simulink model "boatx010"  (R2019b)
settings: Solver=ode4  StartTime=0.0  StopTime=20  FixedStep=0.01  RelTol=1e-3  EnableMultiTasking=on
values from neighbouring files (symbols this model uses):
  A = 10    [sm_boat_runx010.m]
  a1 = a1n(nx)    [sm_boat_runx010.m]
  a2 = a2n(nx)    [sm_boat_runx010.m]
  a3 = a3n(nx)    [sm_boat_runx010.m]
  aa = 50    [sm_boat_runx010.m]
  B = 10    [sm_boat_runx010.m]
  bmax = pi*(0.47)    (= 1.47654854719)    [sm_boat_runx010.m]
  d1 = d1n(nx)    [sm_boat_runx010.m]
  d2 = d2n(nx)    [sm_boat_runx010.m]
  d3 = d3n(nx)    [sm_boat_runx010.m]
  fixedstep = 0.01    [sm_boat_runx010.m]
  Fmax = 20    [sm_boat_runx010.m]
  H = 0.20    (= 0.2)    [sm_boat_runx010.m]
  Iz = m*(W^2+L^2)/12    (= 0.759791666667)    [sm_boat_runx010.m]
  Izz = (0.1*m*W^2+1000*pi*D^2*L^3)/2/12    (= 0.336072151416)    [sm_boat_runx010.m]
  kai = pi*2/8    (= 0.785398163397)    [sm_boat_runx010.m]
  L = 1    [sm_boat_runx010.m]
  Lt = 0.4    [sm_boat_runx010.m]
  m = 7    [sm_boat_runx010.m]
  mxx = 0.05*m    (= 0.35)    [sm_boat_runx010.m]
  myy = 1000*pi*D^2*L/2    (= 3.92699081699)    [sm_boat_runx010.m]
  n_o_w = length(wps)    [sm_boat_runx010.m]
  td = 0    [sm_boat_runx010.m]
  W = 0.55    [sm_boat_runx010.m]
  wd = fd*2*pi    (= 0.628318530718)    [sm_boat_runx010.m]
  wp_sh = 10    [sm_boat_runx010.m]
  wp_tol = 1    [sm_boat_runx010.m]
  wps = [0 0; -aa -aa; aa -aa; aa/2 -aa/2; aa/2 aa/2; aa aa; -aa aa; -aa/2 aa/2; -aa/2 0; -aa/5 0]    [sm_boat_runx010.m]
undefined symbols (not defined in the file or in its folder): X, Y, Z
libraries: sm_lib x36, nesl_utility x11
(part 1 of 2)
settings Model: Creator=huangy  LastModifiedBy=ya
settings DataIOCC: LimitDataPoints=on  SaveFormat=Array  ReturnWorkspaceOutputs=off
settings OptimizationCC: LifeSpan=inf
settings DebuggingCC: SFUnexpectedBacktrackingDiag=warning  SFNoUnconditionalDefaultTransitionDiag=warning  ArithmeticOperatorsInVariantConditions=warning
settings HardwareCC: ProdBitPerPointer=32  ProdBitPerSizeT=32  ProdBitPerPtrDiffT=32  ProdLargestAtomicFloat=None  ProdIntDivRoundTo=Undefined  ProdEndianess=Unspecified  ProdWordSize=32  ProdHWDeviceType=32-bit Generic
settings ModelReferenceCC: PropagateSignalLabelsOutOfModel=off
settings SFSimCC: SimUseLocalCustomCode=off  CustomCodeUndefinedFunction=UseInterfaceOnly
settings RTWCC: RTWUseLocalCustomCode=off
settings CodeAppCC: StateflowObjectComments=on
settings GRTTargetCC: TargetLangStandard=C89/C90 (ANSI)  GeneratePreprocessorConditionals=Disable all
settings ConfigComp: CovMetricSettings=dw  CovHtmlReporting=on  CovSaveCumulativeToWorkspaceVar=on  CovSaveSingleToWorkspaceVar=on  CovExternalEMLEnable=off
settings SimscapeCC: SimscapeNormalizeSystem=off
settings ConfigurationSet: Description=SimMechanics 2G
settings ExplorerConfigSet: InternalSimMechanicsExplorerSettings="<ExplorerConfiguration><canonicalview>default</canonicalview><AnimationSetting><BasePlaybackSpeed>1.0</BasePlaybackSpeed><PlaybackSpeedFactor>1.0</PlaybackSpeedFactor></AnimationSetting><TilePanel><TileInfo><Tiles Columns=\"1\" Count=\"1\" Rows=\"1\"><Column Weight=\"1\"/><Row Weight=\"1\"/><Tile Height=\"1\" Width=\"1\" X=\"0\" Y=\"0\"/></Tiles></TileInfo><SceneInfo><SceneViewer><BGColor><R>0.60000002384185791</R><G>0.60000002384185791</G><B>0.60000002384185791</B></BGColor><Camera><DoPerspective>off</DoPerspective><Position><X>40.4002730296998891</X><Y>-86.2507379862350376</Y><Z>44.8685618917037345</Z></Position><Center><X>-16.7562514385694357</X><Y>-29.0942135179657271</Y><Z>-12.2879625765655653</Z></Center><Up><X>-0.408248290463863073</X><Y>0.408248290463863073</Y><Z>0.816496580927726145</Z></Up><ViewLimDist>1</ViewLimDist><YLim>29.9592729600567189</YLim><XLim>38.3059771851572677</XLim></Camera></SceneViewer></SceneInfo></TilePanel><MechEditorPanel><Cameras/><GfxPanelCameraMap/><VideoCreator><PlaybackSpeedRatio>1.0</PlaybackSpeedRatio><FrameRate>30</FrameRate><VideoFormat>MPEG-4</VideoFormat><FrameSize>[800 600]</FrameSize></VideoCreator></MechEditorPanel></ExplorerConfiguration>"

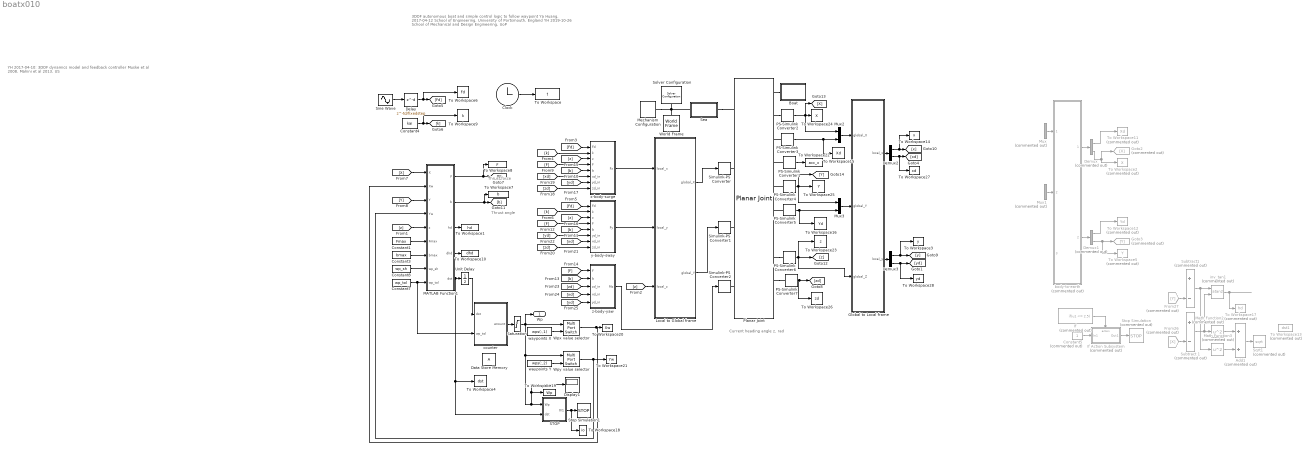
== system boatx010 ==
  note: 3DOF autonomous boat and simple control logic to follow waypoint
      | Ya Huang, 2017-04-12 School of Engineering, University of Portsmouth, England
      | YH 2019-10-26 School of Mechanical and Design Engineering, UoP
  note: Thrust force
  note: Thrust angle
  note: Current heading angle z, rad
  note: YH 2017-04-10:
      | 3DOF dynamics model and feedback controller
      | Muske et al 2008, Mahini et al 2013, US
  Add1 : Sum  Commented=on
  Boat : Subsystem  mask{d=L, w=W, h=H, m=m, Iz=Iz}
      mask prompts: d "Depth d (m)"; w "Width w (m)"; h "Height h (m)"; m "Mass m (kg)"; Iz "Mass moent of inertia"
  Clock : Clock
  Constant1 : Constant  Value=Fmax  VectorParams1D=off
  Constant3 : Constant  Value=bmax  VectorParams1D=off
  Constant4 : Constant  Value=kai
  Constant5 : Constant  Commented=on  VectorParams1D=off
  Constant7 : Constant  Value=wp_tol  VectorParams1D=off
  Constant8 : Constant  Value=wp_sh  VectorParams1D=off
  Data Store Memory : DataStoreMemory  ReadBeforeWriteMsg=warning  WriteAfterWriteMsg=warning  WriteAfterReadMsg=warning  ShowAdditionalParam=off  OutDataTypeStr=single
  Delay : Delay  DelayLength=td/fixedstep  InitialCondition=0
  Demux : Demux  Commented=on  Outputs=2
  Demux1 : Demux  Commented=on  Outputs=2
  Demux2 : Demux  Outputs=2
  Demux3 : Demux  Outputs=2
  Display1 : Display
  From26 : From  Commented=on  GotoTag=X
  From27 : From  Commented=on  GotoTag=Y
  Global to Local frame : Subsystem
  Goto2 : Goto  Commented=on  GotoTag=X
  Goto3 : Goto  Commented=on  GotoTag=Y
  If : If  Commented=on  IfExpression=u1 <= 2.5  ShowElse=off
  If Action Subsystem : Subsystem  Commented=on  TreatAsAtomicUnit=on
  Local to Global frame : Subsystem
  MATLAB Function1 : MATLAB Function  TreatAsAtomicUnit=on
  Math Function2 : Math  Commented=on  Operator=square  SaturateOnIntegerOverflow=on
  Math Function3 : Math  Commented=on  Operator=square  SaturateOnIntegerOverflow=on
  Mechanism Configuration : sm_lib/Utilities/Mechanism Configuration  UniformGravity=Constant  GravityVector=[0 0 -9.80665]  GravityUnits=m/s^2  LinearizationDelta=0.001
  Mux : Mux  Commented=on  Inputs=2
  Mux1 : Mux  Commented=on  Inputs=2
  Mux2 : Mux  Inputs=2
  Mux3 : Mux  Inputs=2
  PS-Simulink Converter1 : nesl_utility/PS-Simulink Converter  PhysicalDomain=network_engine_domain  SubClassName=ps_output  LeftPortType=input  RightPortType=output  PseudoPeriodic=off  Frequencies=[]  Unit=m/s^2  AffineConversion=off
  PS-Simulink Converter2 : nesl_utility/PS-Simulink Converter  PhysicalDomain=network_engine_domain  SubClassName=ps_output  LeftPortType=input  RightPortType=output  PseudoPeriodic=off  Frequencies=[]  Unit=m  AffineConversion=off
  PS-Simulink Converter3 : nesl_utility/PS-Simulink Converter  PhysicalDomain=network_engine_domain  SubClassName=ps_output  LeftPortType=input  RightPortType=output  PseudoPeriodic=off  Frequencies=[]  Unit=m/s  AffineConversion=off
  PS-Simulink Converter4 : nesl_utility/PS-Simulink Converter  PhysicalDomain=network_engine_domain  SubClassName=ps_output  LeftPortType=input  RightPortType=output  PseudoPeriodic=off  Frequencies=[]  Unit=m  AffineConversion=off
  PS-Simulink Converter5 : nesl_utility/PS-Simulink Converter  PhysicalDomain=network_engine_domain  SubClassName=ps_output  LeftPortType=input  RightPortType=output  PseudoPeriodic=off  Frequencies=[]  Unit=m/s  AffineConversion=off
  PS-Simulink Converter6 : nesl_utility/PS-Simulink Converter  PhysicalDomain=network_engine_domain  SubClassName=ps_output  LeftPortType=input  RightPortType=output  PseudoPeriodic=off  Frequencies=[]  Unit=rad  AffineConversion=off
  PS-Simulink Converter7 : nesl_utility/PS-Simulink Converter  PhysicalDomain=network_engine_domain  SubClassName=ps_output  LeftPortType=input  RightPortType=output  PseudoPeriodic=off  Frequencies=[]  Unit=rad/s  AffineConversion=off
  Planar Joint : sm_lib/Joints/Planar Joint  JointMode=Normal  SenseConstraintForce=off  SenseConstraintForceX=off  SenseConstraintForceY=off  SenseConstraintForceZ=off  SenseConstraintTorque=off  SenseConstraintTorqueX=off  SenseConstraintTorqueY=off  SenseConstraintTorqueZ=off  SenseTotalForce=off  SenseTotalForceX=off  SenseTotalForceY=off  SenseTotalForceZ=off  SenseTotalTorque=off  SenseTotalTorqueX=off  SenseTotalTorqueY=off  SenseTotalTorqueZ=off  CompositeWrenchDir=FollowerOnBase  CompositeWrenchFrame=BaseFrame  PxEquilibriumPosition=0  PxEquilibriumPositionUnits=m  PxSpringStiffness=0  PxSpringStiffnessUnits=N/m  PxDampingCoefficient=0  PxDampingCoefficientUnits=N/(m/s)  PxTorqueActuationMode=InputTorque  PxMotionActuationMode=ComputedMotion  PxSensePosition=on  PxSenseVelocity=on  PxSenseAcceleration=on  PxSenseTorqueForce=off  PxSenseLowerLimitTorqueForce=off  PxSenseUpperLimitTorqueForce=off  PxLowerLimitSpecify=off  PxLowerLimitBound=-1  PxLowerLimitBoundUnits=m  PxLowerLimitStiffness=1e6  PxLowerLimitStiffnessUnits=N/m  PxLowerLimitDamping=1e3  PxLowerLimitDampingUnits=N/(m/s)  PxLowerLimitTransitionRegionWidth=1e-4  PxLowerLimitTransitionRegionWidthUnits=m  PxUpperLimitSpecify=off  PxUpperLimitBound=1  PxUpperLimitBoundUnits=m  PxUpperLimitStiffness=1e6  PxUpperLimitStiffnessUnits=N/m  PxUpperLimitDamping=1e3  PxUpperLimitDampingUnits=N/(m/s)  PxUpperLimitTransitionRegionWidth=1e-4  PxUpperLimitTransitionRegionWidthUnits=m  PxPositionTargetSpecify=on  PxPositionTargetPriority=High  PxPositionTargetValue=0  PxPositionTargetValueUnits=m  PxVelocityTargetSpecify=on  PxVelocityTargetPriority=High  PxVelocityTargetValue=0  PxVelocityTargetValueUnits=m/s  PyEquilibriumPosition=0  PyEquilibriumPositionUnits=m  PySpringStiffness=0  PySpringStiffnessUnits=N/m  PyDampingCoefficient=0  PyDampingCoefficientUnits=N/(m/s)  PyTorqueActuationMode=InputTorque  PyMotionActuationMode=ComputedMotion  PySensePosition=on  PySenseVelocity=on  PySenseAcceleration=on  PySenseTorqueForce=off  PySenseLowerLimitTorqueForce=off  PySenseUpperLimitTorqueForce=off  PyLowerLimitSpecify=off  PyLowerLimitBound=-1  PyLowerLimitBoundUnits=m  PyLowerLimitStiffness=1e6  PyLowerLimitStiffnessUnits=N/m  PyLowerLimitDamping=1e3  PyLowerLimitDampingUnits=N/(m/s)  PyLowerLimitTransitionRegionWidth=1e-4  PyLowerLimitTransitionRegionWidthUnits=m  PyUpperLimitSpecify=off  PyUpperLimitBound=1  PyUpperLimitBoundUnits=m  PyUpperLimitStiffness=1e6  PyUpperLimitStiffnessUnits=N/m  PyUpperLimitDamping=1e3  PyUpperLimitDampingUnits=N/(m/s)  PyUpperLimitTransitionRegionWidth=1e-4  PyUpperLimitTransitionRegionWidthUnits=m  PyPositionTargetSpecify=on  PyPositionTargetPriority=High  PyPositionTargetValue=0  PyPositionTargetValueUnits=m  PyVelocityTargetSpecify=on  PyVelocityTargetPriority=High  PyVelocityTargetValue=0  PyVelocityTargetValueUnits=m/s  RzEquilibriumPosition=0  RzEquilibriumPositionUnits=deg  RzSpringStiffness=0  RzSpringStiffnessUnits=N*m/deg  RzDampingCoefficient=0  RzDampingCoefficientUnits=N*m/(deg/s)  RzTorqueActuationMode=InputTorque  RzMotionActuationMode=ComputedMotion  RzSensePosition=on  RzSenseVelocity=on  RzSenseAcceleration=on  RzSenseTorqueForce=off  RzSenseLowerLimitTorqueForce=off  RzSenseUpperLimitTorqueForce=off  RzLowerLimitSpecify=off  RzLowerLimitBound=-90  RzLowerLimitBoundUnits=deg  RzLowerLimitStiffness=1e4  RzLowerLimitStiffnessUnits=N*m/deg  RzLowerLimitDamping=10  RzLowerLimitDampingUnits=N*m/(deg/s)  RzLowerLimitTransitionRegionWidth=0.1  RzLowerLimitTransitionRegionWidthUnits=deg  RzUpperLimitSpecify=off  RzUpperLimitBound=90  RzUpperLimitBoundUnits=deg  RzUpperLimitStiffness=1e4  RzUpperLimitStiffnessUnits=N*m/deg  RzUpperLimitDamping=10  RzUpperLimitDampingUnits=N*m/(deg/s)  RzUpperLimitTransitionRegionWidth=0.1  RzUpperLimitTransitionRegionWidthUnits=deg  RzPositionTargetSpecify=on  RzPositionTargetPriority=High  RzPositionTargetValue=0  RzPositionTargetValueUnits=deg  RzVelocityTargetSpecify=on  RzVelocityTargetPriority=High  RzVelocityTargetValue=0  RzVelocityTargetValueUnits=deg/s
  STOP : Subsystem
  Saturation : Saturate  UpperLimit=n_o_w  LowerLimit=0  OutDataTypeStr=double
  Sea : Subsystem  mask{d=100, w=100, h=0.1, rho=0}
      mask prompts: d "Depth d (m)"; w "Width w (m)"; h "Height h (m)"; rho "Density rho (kg/m^3)"
  Simulink-PS Converter : nesl_utility/Simulink-PS Converter  PhysicalDomain=network_engine_domain  SubClassName=ps_input  LeftPortType=input  RightPortType=output  PseudoPeriodic=off  Frequencies=[]  NoiseDistribution=none  NoiseParameters=[]  Unit=N  AffineConversion=off  FilteringAndDerivatives=zero  SimscapeFilterOrder=1  InputFilterTimeConstant=0.001  UdotUserProvided=1
  Simulink-PS Converter1 : nesl_utility/Simulink-PS Converter  PhysicalDomain=network_engine_domain  SubClassName=ps_input  LeftPortType=input  RightPortType=output  PseudoPeriodic=off  Frequencies=[]  NoiseDistribution=none  NoiseParameters=[]  Unit=N  AffineConversion=off  FilteringAndDerivatives=zero  SimscapeFilterOrder=1  InputFilterTimeConstant=0.001  UdotUserProvided=1
  Simulink-PS Converter2 : nesl_utility/Simulink-PS Converter  PhysicalDomain=network_engine_domain  SubClassName=ps_input  LeftPortType=input  RightPortType=output  PseudoPeriodic=off  Frequencies=[]  NoiseDistribution=none  NoiseParameters=[]  Unit=N*m  AffineConversion=off  FilteringAndDerivatives=zero  SimscapeFilterOrder=1  InputFilterTimeConstant=0.001  UdotUserProvided=1
  Sine Wave : Sin  Amplitude=A  Bias=B  Frequency=wd  SampleTime=0
  Solver Configuration : nesl_utility/Solver Configuration  PhysicalDomain=network_engine_domain  SubClassName=solver  LeftPortType=input  RightPortType=generic  Tones=[]  Harmonics=[]  SimulateNoise=off  Profile=off  UseLocalSampling=off  EnableSwitchedLinearOptims=on  FrequencyDomain=off  UseCCode=off  RelTol=0.001  AbsTol=1e-06  MinStep=1e-09  ToWorkspace=off  RevertToSquareIcSolve=off  NumHomotopyIterations=100  PhasorMode=off  PhasorModeNumHarmonics=1  DoDC=off  ResidualTolerance=1e-09  UseLocalSolver=off  LocalSolverChoice=NE_BACKWARD_EULER_ADVANCER  LocalSolverSampleTime=0.001  DoFixedCost=off  MaxNonlinIter=3  MaxModeIter=2  LinearAlgebra=Sparse  EquationFormulation=NE_TIME_EF  DelaysMemoryBudget=1024  AutomaticFiltering=on  FilteringTimeConstant=0.001  PartitionStorageMethod=AS_NEEDED  PartitionMemoryBudget=1024  PartitionMethod=FAST
  Sqrt1 : Sqrt  Commented=on  SaturateOnIntegerOverflow=on
  Stop Simulation : Stop  Commented=on
  Stop Simulation1 : Stop
  Subtract 1 : Sum  Commented=on  Inputs=+-
  Subtract1 : Sum  Commented=on  Inputs=+-
  To Workspace : ToWorkspace  VariableName=t  SaveFormat=Timeseries  SampleTime=-1
  To Workspace1 : ToWorkspace  VariableName=hd  SaveFormat=Timeseries  SampleTime=-1
  To Workspace10 : ToWorkspace  VariableName=dhd  SaveFormat=Timeseries  SampleTime=-1
  To Workspace11 : ToWorkspace  Commented=on  VariableName=Xd  SaveFormat=Timeseries  SampleTime=-1
  To Workspace12 : ToWorkspace  Commented=on  VariableName=Yd  SaveFormat=Timeseries  SampleTime=-1
  To Workspace13 : ToWorkspace  Commented=on  VariableName=dst1  SaveFormat=Timeseries  SampleTime=-1
  To Workspace14 : ToWorkspace  VariableName=x  SaveFormat=Timeseries  SampleTime=-1
  To Workspace15 : ToWorkspace  VariableName=Xd  SaveFormat=Timeseries  SampleTime=-1
      settings: Save2DSignal=2-D array (concatenate along first dimension)
  To Workspace16 : ToWorkspace  VariableName=Yd  SaveFormat=Timeseries  SampleTime=-1
  To Workspace17 : ToWorkspace  Commented=on  VariableName=hd  SaveFormat=Timeseries  SampleTime=-1
  To Workspace18 : ToWorkspace  VariableName=io  SaveFormat=Timeseries  SampleTime=-1
  To Workspace19 : ToWorkspace  VariableName=Wp  SaveFormat=Timeseries  SampleTime=-1
  To Workspace2 : ToWorkspace  Commented=on  VariableName=X  SaveFormat=Timeseries  SampleTime=-1
  To Workspace20 : ToWorkspace  VariableName=Xw  SaveFormat=Timeseries  SampleTime=-1
  To Workspace21 : ToWorkspace  VariableName=Yw  SaveFormat=Timeseries  SampleTime=-1
  To Workspace22 : ToWorkspace  VariableName=acc_x  SaveFormat=Timeseries  SampleTime=-1
      settings: Save2DSignal=2-D array (concatenate along first dimension)
  To Workspace23 : ToWorkspace  VariableName=z  SaveFormat=Timeseries  SampleTime=-1
  To Workspace24 : ToWorkspace  VariableName=X  SaveFormat=Timeseries  SampleTime=-1
      settings: Save2DSignal=2-D array (concatenate along first dimension)
  To Workspace25 : ToWorkspace  VariableName=Y  SaveFormat=Timeseries  SampleTime=-1
  To Workspace26 : ToWorkspace  VariableName=zd  SaveFormat=Timeseries  SampleTime=-1
  To Workspace27 : ToWorkspace  VariableName=xd  SaveFormat=Timeseries  SampleTime=-1
  To Workspace28 : ToWorkspace  VariableName=yd  SaveFormat=Timeseries  SampleTime=-1
  To Workspace3 : ToWorkspace  VariableName=y  SaveFormat=Timeseries  SampleTime=-1
  To Workspace4 : ToWorkspace  VariableName=dst  SaveFormat=Timeseries  SampleTime=-1
  To Workspace5 : ToWorkspace  Commented=on  VariableName=Y  SaveFormat=Timeseries  SampleTime=-1
  To Workspace6 : ToWorkspace  VariableName=Fd  SaveFormat=Timeseries  SampleTime=-1
  To Workspace7 : ToWorkspace  VariableName=b  SaveFormat=Timeseries  SampleTime=-1
  To Workspace8 : ToWorkspace  VariableName=F  SaveFormat=Timeseries  SampleTime=-1
  To Workspace9 : ToWorkspace  VariableName=k  SaveFormat=Timeseries  SampleTime=-1
  Unit Delay : UnitDelay  SampleTime=-1  HasFrameUpgradeWarning=on
  World Frame : sm_lib/Frames and Transforms/World Frame
  Wpx value selector : MultiPortSwitch  Inputs=1
  Wpy value selector : MultiPortSwitch  Inputs=1
  body-to-earth : Subsystem  Commented=on
  counter : MATLAB Function  TreatAsAtomicUnit=on
  inv_tan1 : Trigonometry  Commented=on  Operator=atan2  OutputSignalType=real
  waypoints X : Constant  Value=wps(:,1)
  waypoints Y : Constant  Value=wps(:,2)
  x-body-surge : Subsystem
  y-body-sway : Subsystem
  z-body-yaw : Subsystem
  Wp : Outport  OutDataTypeStr=double  VectorParamsAs1DForOutWhenUnconnected=off
  wires:
  Clock/1 -> To Workspace/1
  [X] -> MATLAB Function1/1(X)
  [Y] -> MATLAB Function1/3(Y)
  [z] -> MATLAB Function1/5(z)
  Constant1/1 -> MATLAB Function1/6(Fmax)
  Constant3/1 -> MATLAB Function1/7(bmax)
  MATLAB Function1/3(hd) -> To Workspace1/1
  Constant4/1 -> To Workspace9/1, [k]
  [Fd] -> x-body-surge/1(Fd)
  [k] -> x-body-surge/2(k)
  [Fd] -> y-body-sway/1(Fd)
  [k] -> y-body-sway/2(k)
  [F] -> x-body-surge/4(F)
  [b] -> x-body-surge/5(b)
  [b] -> y-body-sway/5(b)
  [F] -> y-body-sway/4(F)
  [F] -> z-body-yaw/1(F)
  [b] -> z-body-yaw/2(b)
  [z] -> x-body-surge/3(z)
  [z] -> y-body-sway/3(z)
  Sine Wave/1 -> Delay/1
  Delay/1 -> [Fd], To Workspace6/1
  If/1 -> If Action Subsystem/Action
  If Action Subsystem/1(Out1) -> Stop Simulation/1
  Constant5/1 -> If Action Subsystem/1(In1)
  Constant8/1 -> MATLAB Function1/8(wp_sh)
  [yd] -> x-body-surge/7(yd_in)
  [zd] -> x-body-surge/8(zd_in)
  [xd] -> x-body-surge/6(xd_in)
  [yd] -> y-body-sway/6(yd_in)
  [zd] -> y-body-sway/8(zd_in)
  [xd] -> y-body-sway/7(xd_in)
  [zd] -> z-body-yaw/3(zd_in)
  [xd] -> z-body-yaw/4(xd_in)
  [yd] -> z-body-yaw/5(yd_in)
  Mux/1 -> body-to-earth/1(x_body)
  Mux1/1 -> body-to-earth/2(y_body)
  body-to-earth/1(X_earth) -> Demux/1
  body-to-earth/2(Y_earth) -> Demux1/1
  Demux1/2 -> To Workspace5/1, Goto3/1
  Demux/2 -> Goto2/1, To Workspace2/1
  Demux/1 -> To Workspace11/1
  Demux1/1 -> To Workspace12/1
  Add1/1 -> Sqrt1/1
  waypoints Y/1 -> Wpy value selector/2
  Subtract 1/1 -> inv_tan1/2, Math Function2/1
  From26/1 -> Subtract 1/2
  Math Function2/1 -> Add1/1
  From27/1 -> Subtract1/2
  waypoints X/1 -> Wpx value selector/2
  Math Function3/1 -> Add1/2
  Subtract1/1 -> Math Function3/1, inv_tan1/1
  inv_tan1/1 -> To Workspace17/1
  counter/1(wcount) -> Saturation/1
  Constant7/1 -> counter/2(wp_tol), MATLAB Function1/9(wp_tol)
  MATLAB Function1/5(dst) -> STOP/2(dst), To Workspace4/1, Unit Delay/1
  Wpx value selector/1 -> MATLAB Function1/2(Xw), To Workspace20/1
  Wpy value selector/1 -> To Workspace21/1, MATLAB Function1/4(Yw)
  Saturation/1 -> STOP/1(Wp), To Workspace19/1, Display1/1, Wpy value selector/1, Wp/1, Wpx value selector/1
  STOP/1(0/1) -> To Workspace18/1, Stop Simulation1/1
  Unit Delay/1 -> counter/1(dst)
  MATLAB Function1/1(F) -> [F], To Workspace8/1
  PS-Simulink Converter4/1 -> To Workspace25/1, [Y], Mux3/1
  PS-Simulink Converter1/1 -> To Workspace22/1
  PS-Simulink Converter6/1 -> [z], Global to Local frame/3(global_Z), To Workspace23/1
  PS-Simulink Converter2/1 -> Mux2/1, [X], To Workspace24/1
  z-body-yaw/1(Mz) -> Simulink-PS Converter2/1
  Mux2/1 -> Global to Local frame/1(global_X)
  PS-Simulink Converter3/1 -> To Workspace15/1, Mux2/2
  Mux3/1 -> Global to Local frame/2(global_Y)
  PS-Simulink Converter5/1 -> Mux3/2, To Workspace16/1
  Global to Local frame/1(local_x) -> Demux2/1
  Global to Local frame/2(local_y) -> Demux3/1
  [z] -> Local to Global frame/3(local_z)
  x-body-surge/1(Fx) -> Local to Global frame/1(local_x)
  y-body-sway/1(Fy) -> Local to Global frame/2(local_y)
  Local to Global frame/1(global_X) -> Simulink-PS Converter/1
  Local to Global frame/2(global_Y) -> Simulink-PS Converter1/1
  PS-Simulink Converter7/1 -> [zd], To Workspace26/1
  Demux3/2 -> To Workspace28/1, [yd]
  Demux3/1 -> To Workspace3/1, [y]
  Demux2/1 -> To Workspace14/1, [x]
  Demux2/2 -> To Workspace27/1, [xd]
  MATLAB Function1/4(dhd) -> To Workspace10/1
  MATLAB Function1/2(b) -> To Workspace7/1, [b]
  connections:
  Planar Joint/RConn8 -- PS-Simulink Converter6/LConn1
  Planar Joint/RConn9 -- PS-Simulink Converter7/LConn1
  Simulink-PS Converter2/RConn1 -- Planar Joint/LConn4
  Sea/RConn1 -- Planar Joint/LConn1
  Planar Joint/RConn2 -- PS-Simulink Converter2/LConn1
  Planar Joint/RConn1 -- Boat/LConn1
  PS-Simulink Converter3/LConn1 -- Planar Joint/RConn3
  PS-Simulink Converter4/LConn1 -- Planar Joint/RConn5
  PS-Simulink Converter5/LConn1 -- Planar Joint/RConn6
  PS-Simulink Converter1/LConn1 -- Planar Joint/RConn4
  Solver Configuration/RConn1 -- World Frame/RConn1 -- Mechanism Configuration/RConn1 -- Sea/LConn1
  Simulink-PS Converter/RConn1 -- Planar Joint/LConn2
  Simulink-PS Converter1/RConn1 -- Planar Joint/LConn3

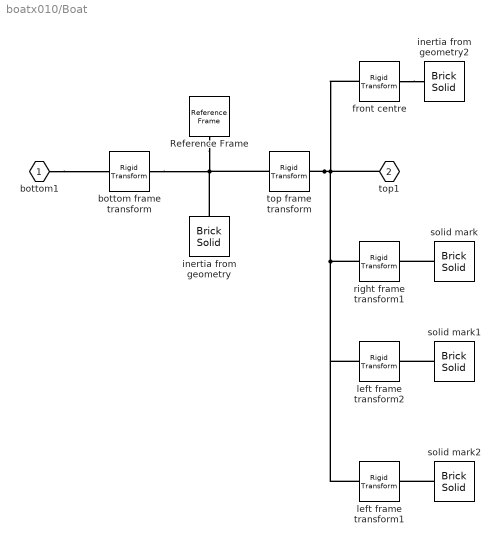
== system boatx010/Boat ==
  Reference Frame : sm_lib/Frames and Transforms/Reference Frame
  bottom frame transform : sm_lib/Frames and Transforms/Rigid Transform  TranslationMethod=StandardAxis  TranslationStandardOffset=h  TranslationLengthUnit=m  TranslationStandardAxis=-Z  TranslationCartesianOffset=[0 0 -h/2]  TranslationROffset=0  TranslationROffsetUnits=m  TranslationZOffset=0  TranslationZOffsetUnits=m  TranslationThetaOffset=0  TranslationThetaOffsetUnits=deg  RotationMethod=None  RotationAngleUnits=deg  RotationStandardAxis=+Z  RotationAngle=0  RotationArbitraryAxis=[0 0 1]  FollAlignAxisA=+Y  BaseAlignAxisA=-Z  FollAlignAxisB=+Z  BaseAlignAxisB=-X  RotationSequenceAxes=FollowerAxes  RotationSequence=XYX  RotationSequenceAngles=[0 0 0]  RotationSequenceAnglesUnits=deg  RotationMatrix=[1 0 0; 0 1 0; 0 0 1]
  front centre : sm_lib/Frames and Transforms/Rigid Transform  TranslationMethod=Cartesian  TranslationStandardOffset=w/2  TranslationLengthUnit=m  TranslationStandardAxis=+Y  TranslationCartesianOffset=[d/2+h/2 0 -h/2]  TranslationROffset=0  TranslationROffsetUnits=m  TranslationZOffset=0  TranslationZOffsetUnits=m  TranslationThetaOffset=0  TranslationThetaOffsetUnits=deg  RotationMethod=None  RotationAngleUnits=deg  RotationStandardAxis=+Z  RotationAngle=0  RotationArbitraryAxis=[0 0 1]  FollAlignAxisA=+Z  BaseAlignAxisA=-X  FollAlignAxisB=+X  BaseAlignAxisB=+Y  RotationSequenceAxes=FollowerAxes  RotationSequence=XYX  RotationSequenceAngles=[0 0 0]  RotationSequenceAnglesUnits=deg  RotationMatrix=[1 0 0; 0 1 0; 0 0 1]
  inertia from geometry : sm_lib/Body Elements/Brick Solid  GraphicAmbientColor=[0.15 0.15 0.15 1.0]  BasedOnType=Density  BrickDimensions=[d w h]  BrickDimensionUnits=m  CenterOfMass=[0 0 0]  CenterOfMassUnits=m  GraphicDiffuseColor=[1.0 1.0 0.0]  Density=900  DensityUnits=kg/(m^3)  DoExposeReferenceFrame=on  GraphicEmissiveColor=[0.0 0.0 0.0 1.0]  ExportEntireGeometry=off  SerializedFrames=<Frames/>  MarkerShape=Sphere  MarkerSize=10  GraphicType=FromGeometry  InertiaType=Custom  Mass=m  MassUnits=kg  MomentsOfInertia=[0 0 Iz]  MomentsOfInertiaUnits=kg*m^2  GraphicOpacity=0.8  ProductsOfInertia=[0 0 0]  ProductsOfInertiaUnits=kg*m^2  GraphicShininess=75  GraphicSpecularColor=[0.5 0.5 0.5 1.0]  GraphicVisPropType=SimpleVisualProperties
  inertia from geometry2 : sm_lib/Body Elements/Brick Solid  GraphicAmbientColor=[0.15 0.15 0.15 1.0]  BasedOnType=Density  BrickDimensions=[h h h]  BrickDimensionUnits=m  CenterOfMass=[d/2 w/2 h/2]  CenterOfMassUnits=m  GraphicDiffuseColor=[1.0 1.0 0.0]  Density=900  DensityUnits=kg/(m^3)  DoExposeReferenceFrame=on  GraphicEmissiveColor=[0.0 0.0 0.0 1.0]  ExportEntireGeometry=off  SerializedFrames=<Frames/>  MarkerShape=Sphere  MarkerSize=10  GraphicType=FromGeometry  InertiaType=PointMass  Mass=0  MassUnits=kg  MomentsOfInertia=[1 1 Izz]  MomentsOfInertiaUnits=kg*m^2  GraphicOpacity=0.8  ProductsOfInertia=[0 0 0]  ProductsOfInertiaUnits=kg*m^2  GraphicShininess=75  GraphicSpecularColor=[0.5 0.5 0.5 1.0]  GraphicVisPropType=SimpleVisualProperties
  left frame transform1 : sm_lib/Frames and Transforms/Rigid Transform  TranslationMethod=Cartesian  TranslationStandardOffset=w/2  TranslationLengthUnit=m  TranslationStandardAxis=+Y  TranslationCartesianOffset=[-d/2 w/2 0]  TranslationROffset=0  TranslationROffsetUnits=m  TranslationZOffset=0  TranslationZOffsetUnits=m  TranslationThetaOffset=0  TranslationThetaOffsetUnits=deg  RotationMethod=None  RotationAngleUnits=deg  RotationStandardAxis=+Z  RotationAngle=0  RotationArbitraryAxis=[0 0 1]  FollAlignAxisA=+Z  BaseAlignAxisA=-X  FollAlignAxisB=+X  BaseAlignAxisB=+Y  RotationSequenceAxes=FollowerAxes  RotationSequence=XYX  RotationSequenceAngles=[0 0 0]  RotationSequenceAnglesUnits=deg  RotationMatrix=[1 0 0; 0 1 0; 0 0 1]
  left frame transform2 : sm_lib/Frames and Transforms/Rigid Transform  TranslationMethod=Cartesian  TranslationStandardOffset=w/2  TranslationLengthUnit=m  TranslationStandardAxis=+Y  TranslationCartesianOffset=[-d/2 -w/2 0]  TranslationROffset=0  TranslationROffsetUnits=m  TranslationZOffset=0  TranslationZOffsetUnits=m  TranslationThetaOffset=0  TranslationThetaOffsetUnits=deg  RotationMethod=None  RotationAngleUnits=deg  RotationStandardAxis=+Z  RotationAngle=0  RotationArbitraryAxis=[0 0 1]  FollAlignAxisA=+Z  BaseAlignAxisA=-X  FollAlignAxisB=+X  BaseAlignAxisB=+Y  RotationSequenceAxes=FollowerAxes  RotationSequence=XYX  RotationSequenceAngles=[0 0 0]  RotationSequenceAnglesUnits=deg  RotationMatrix=[1 0 0; 0 1 0; 0 0 1]
  right frame transform1 : sm_lib/Frames and Transforms/Rigid Transform  TranslationMethod=Cartesian  TranslationStandardOffset=w/2  TranslationLengthUnit=m  TranslationStandardAxis=+Y  TranslationCartesianOffset=[-d/2-h/2/2 0 -h]  TranslationROffset=0  TranslationROffsetUnits=m  TranslationZOffset=0  TranslationZOffsetUnits=m  TranslationThetaOffset=0  TranslationThetaOffsetUnits=deg  RotationMethod=None  RotationAngleUnits=deg  RotationStandardAxis=+Z  RotationAngle=0  RotationArbitraryAxis=[0 0 1]  FollAlignAxisA=+Z  BaseAlignAxisA=-X  FollAlignAxisB=+X  BaseAlignAxisB=+Y  RotationSequenceAxes=FollowerAxes  RotationSequence=XYX  RotationSequenceAngles=[0 0 0]  RotationSequenceAnglesUnits=deg  RotationMatrix=[1 0 0; 0 1 0; 0 0 1]
  solid mark : sm_lib/Body Elements/Brick Solid  GraphicAmbientColor=[0.15 0.15 0.15 1.0]  BasedOnType=Density  BrickDimensions=[h/2 h/2 h/2]  BrickDimensionUnits=m  CenterOfMass=[d/2 w/2 h/2]  CenterOfMassUnits=m  GraphicDiffuseColor=[1.0 0.6 0.0]  Density=900  DensityUnits=kg/(m^3)  DoExposeReferenceFrame=on  GraphicEmissiveColor=[0.0 0.0 0.0 1.0]  ExportEntireGeometry=off  SerializedFrames=<Frames/>  MarkerShape=Sphere  MarkerSize=10  GraphicType=FromGeometry  InertiaType=PointMass  Mass=0  MassUnits=kg  MomentsOfInertia=[1 1 Izz]  MomentsOfInertiaUnits=kg*m^2  GraphicOpacity=1  ProductsOfInertia=[0 0 0]  ProductsOfInertiaUnits=kg*m^2  GraphicShininess=75  GraphicSpecularColor=[0.5 0.5 0.5 1.0]  GraphicVisPropType=SimpleVisualProperties
  solid mark1 : sm_lib/Body Elements/Brick Solid  GraphicAmbientColor=[0.15 0.15 0.15 1.0]  BasedOnType=Density  BrickDimensions=[h/2 h/2 h/2]  BrickDimensionUnits=m  CenterOfMass=[d/2 w/2 h/2]  CenterOfMassUnits=m  GraphicDiffuseColor=[0 1 0]  Density=900  DensityUnits=kg/(m^3)  DoExposeReferenceFrame=on  GraphicEmissiveColor=[0.0 0.0 0.0 1.0]  ExportEntireGeometry=off  SerializedFrames=<Frames/>  MarkerShape=Sphere  MarkerSize=10  GraphicType=FromGeometry  InertiaType=PointMass  Mass=0  MassUnits=kg  MomentsOfInertia=[1 1 Izz]  MomentsOfInertiaUnits=kg*m^2  GraphicOpacity=1  ProductsOfInertia=[0 0 0]  ProductsOfInertiaUnits=kg*m^2  GraphicShininess=75  GraphicSpecularColor=[0.5 0.5 0.5 1.0]  GraphicVisPropType=SimpleVisualProperties
  solid mark2 : sm_lib/Body Elements/Brick Solid  GraphicAmbientColor=[0.15 0.15 0.15 1.0]  BasedOnType=Density  BrickDimensions=[h/2 h/2 h/2]  BrickDimensionUnits=m  CenterOfMass=[d/2 w/2 h/2]  CenterOfMassUnits=m  GraphicDiffuseColor=[1.0 0.0 0.0]  Density=900  DensityUnits=kg/(m^3)  DoExposeReferenceFrame=on  GraphicEmissiveColor=[0.0 0.0 0.0 1.0]  ExportEntireGeometry=off  SerializedFrames=<Frames/>  MarkerShape=Sphere  MarkerSize=10  GraphicType=FromGeometry  InertiaType=PointMass  Mass=0  MassUnits=kg  MomentsOfInertia=[1 1 Izz]  MomentsOfInertiaUnits=kg*m^2  GraphicOpacity=1  ProductsOfInertia=[0 0 0]  ProductsOfInertiaUnits=kg*m^2  GraphicShininess=75  GraphicSpecularColor=[0.5 0.5 0.5 1.0]  GraphicVisPropType=SimpleVisualProperties
  top frame transform : sm_lib/Frames and Transforms/Rigid Transform  TranslationMethod=StandardAxis  TranslationStandardOffset=h/2  TranslationLengthUnit=m  TranslationStandardAxis=+Z  TranslationCartesianOffset=[0 0 0]  TranslationROffset=0  TranslationROffsetUnits=m  TranslationZOffset=0  TranslationZOffsetUnits=m  TranslationThetaOffset=0  TranslationThetaOffsetUnits=deg  RotationMethod=None  RotationAngleUnits=deg  RotationStandardAxis=+Z  RotationAngle=0  RotationArbitraryAxis=[0 0 1]  FollAlignAxisA=+Z  BaseAlignAxisA=-X  FollAlignAxisB=+X  BaseAlignAxisB=+Y  RotationSequenceAxes=FollowerAxes  RotationSequence=XYX  RotationSequenceAngles=[0 0 0]  RotationSequenceAnglesUnits=deg  RotationMatrix=[1 0 0; 0 1 0; 0 0 1]
  bottom1 : PMIOPort  Side=Left
  top1 : PMIOPort  Port=2  Side=Right
  connections:
  bottom frame transform/LConn1 -- inertia from geometry/RConn1 -- Reference Frame/RConn1 -- top frame transform/LConn1
  top frame transform/RConn1 -- front centre/LConn1 -- right frame transform1/LConn1 -- left frame transform2/LConn1 -- left frame transform1/LConn1 -- top1/RConn1
  bottom1/RConn1 -- bottom frame transform/RConn1
  solid mark/RConn1 -- right frame transform1/RConn1
  solid mark1/RConn1 -- left frame transform2/RConn1
  solid mark2/RConn1 -- left frame transform1/RConn1
  front centre/RConn1 -- inertia from geometry2/RConn1

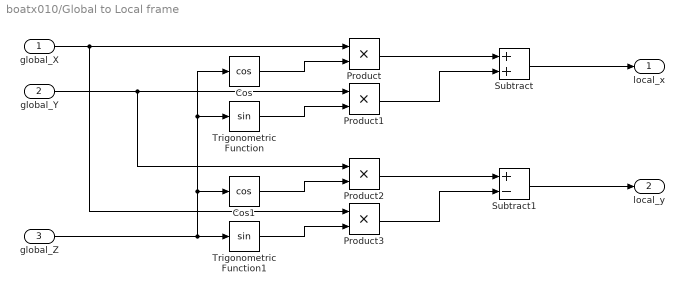
== system boatx010/Global to Local frame ==
  global_X : Inport
  global_Y : Inport  Port=2
  global_Z : Inport  Port=3
  Cos : Trigonometry  Operator=cos
  Cos1 : Trigonometry  Operator=cos
  Product{,1..3} (4 alike) : Product
  Subtract : Sum
  Subtract1 : Sum  Inputs=+-
  Trigonometric Function : Trigonometry
  Trigonometric Function1 : Trigonometry
  local_x : Outport  VectorParamsAs1DForOutWhenUnconnected=off
  local_y : Outport  Port=2  VectorParamsAs1DForOutWhenUnconnected=off
  wires:
  Subtract1/1 -> local_y/1
  Subtract/1 -> local_x/1
  Product/1 -> Subtract/1
  Product2/1 -> Subtract1/1
  Product1/1 -> Subtract/2
  Product3/1 -> Subtract1/2
  global_X/1 -> Product3/1, Product/1
  global_Y/1 -> Product2/1, Product1/1
  global_Z/1 -> Cos1/1, Trigonometric Function/1, Cos/1, Trigonometric Function1/1
  Trigonometric Function1/1 -> Product3/2
  Cos1/1 -> Product2/2
  Trigonometric Function/1 -> Product1/2
  Cos/1 -> Product/2

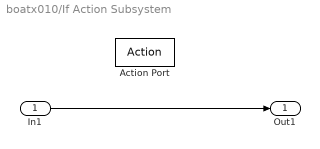
== system boatx010/If Action Subsystem ==
  In1 : Inport
  Action Port : ActionPort  ActionPortLabel=if(u1 <= 2.5)
  Out1 : Outport  VectorParamsAs1DForOutWhenUnconnected=off
  wires:
  In1/1 -> Out1/1

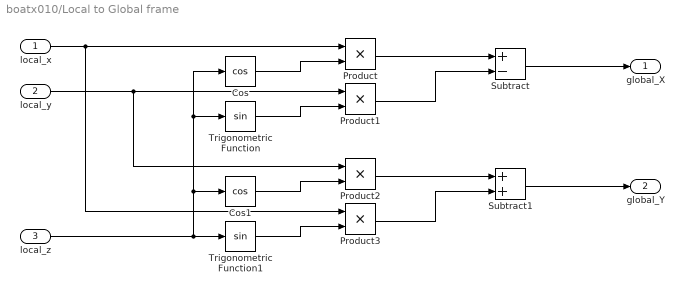
== system boatx010/Local to Global frame ==
  local_x : Inport
  local_y : Inport  Port=2
  local_z : Inport  Port=3
  Cos : Trigonometry  Operator=cos
  Cos1 : Trigonometry  Operator=cos
  Product{,1..3} (4 alike) : Product
  Subtract : Sum  Inputs=+-
  Subtract1 : Sum
  Trigonometric Function : Trigonometry
  Trigonometric Function1 : Trigonometry
  global_X : Outport  VectorParamsAs1DForOutWhenUnconnected=off
  global_Y : Outport  Port=2  VectorParamsAs1DForOutWhenUnconnected=off
  wires:
  Subtract1/1 -> global_Y/1
  Subtract/1 -> global_X/1
  Product/1 -> Subtract/1
  Product2/1 -> Subtract1/1
  Product1/1 -> Subtract/2
  Product3/1 -> Subtract1/2
  local_x/1 -> Product3/1, Product/1
  local_y/1 -> Product2/1, Product1/1
  local_z/1 -> Cos1/1, Trigonometric Function/1, Cos/1, Trigonometric Function1/1
  Trigonometric Function1/1 -> Product3/2
  Cos1/1 -> Product2/2
  Trigonometric Function/1 -> Product1/2
  Cos/1 -> Product/2

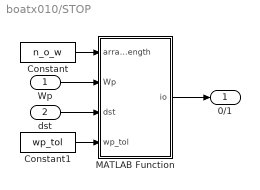
== system boatx010/STOP ==
  Wp : Inport
  dst : Inport  Port=2
  Constant : Constant  Value=n_o_w
  Constant1 : Constant  Value=wp_tol
  MATLAB Function : MATLAB Function  TreatAsAtomicUnit=on
  0/1 : Outport  VectorParamsAs1DForOutWhenUnconnected=off
  wires:
  MATLAB Function/1(io) -> 0/1/1
  Wp/1 -> MATLAB Function/2(Wp)
  dst/1 -> MATLAB Function/3(dst)
  Constant/1 -> MATLAB Function/1(arrayLength)
  Constant1/1 -> MATLAB Function/4(wp_tol)

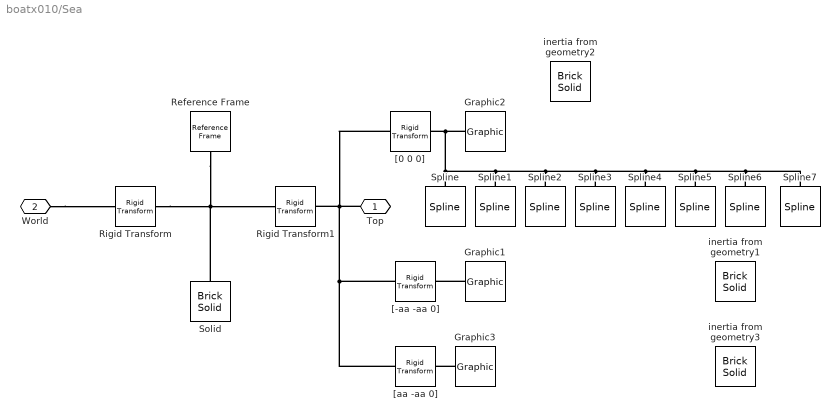
== system boatx010/Sea ==
  Graphic1 : sm_lib/Body Elements/Graphic  GraphicType=Marker  MarkerShape=Cube  MarkerSize=10  GraphicVisPropType=SimpleVisualProperties  GraphicDiffuseColor=[0.6 0.4 0.0]  GraphicSpecularColor=[0.5 0.5 0.5 1.0]  GraphicAmbientColor=[0.15 0.15 0.15 1.0]  GraphicEmissiveColor=[0.0 0.0 0.0 1.0]  GraphicShininess=75  GraphicOpacity=1
      settings: SourceProductName=Simscape Multibody
  Graphic2 : sm_lib/Body Elements/Graphic  GraphicType=Marker  MarkerShape=Cube  MarkerSize=10  GraphicVisPropType=SimpleVisualProperties  GraphicDiffuseColor=[0.6 0.4 0.0]  GraphicSpecularColor=[0.5 0.5 0.5 1.0]  GraphicAmbientColor=[0.15 0.15 0.15 1.0]  GraphicEmissiveColor=[0.0 0.0 0.0 1.0]  GraphicShininess=75  GraphicOpacity=1
      settings: SourceProductName=Simscape Multibody
  Graphic3 : sm_lib/Body Elements/Graphic  GraphicType=Marker  MarkerShape=Cube  MarkerSize=10  GraphicVisPropType=SimpleVisualProperties  GraphicDiffuseColor=[0.6 0.4 0.0]  GraphicSpecularColor=[0.5 0.5 0.5 1.0]  GraphicAmbientColor=[0.15 0.15 0.15 1.0]  GraphicEmissiveColor=[0.0 0.0 0.0 1.0]  GraphicShininess=75  GraphicOpacity=1
      settings: SourceProductName=Simscape Multibody
  Reference Frame : sm_lib/Frames and Transforms/Reference Frame
  Rigid Transform : sm_lib/Frames and Transforms/Rigid Transform  TranslationMethod=StandardAxis  TranslationStandardOffset=h/2  TranslationLengthUnit=m  TranslationStandardAxis=-Z  TranslationCartesianOffset=[0 0 0]  TranslationROffset=0  TranslationROffsetUnits=m  TranslationZOffset=0  TranslationZOffsetUnits=m  TranslationThetaOffset=0  TranslationThetaOffsetUnits=deg  RotationMethod=None  RotationAngleUnits=deg  RotationStandardAxis=+Z  RotationAngle=0.0  RotationArbitraryAxis=[0 0 1]  FollAlignAxisA=+X  BaseAlignAxisA=+Y  FollAlignAxisB=+Y  BaseAlignAxisB=+Z  RotationSequenceAxes=FollowerAxes  RotationSequence=XYX  RotationSequenceAngles=[0 0 0]  RotationSequenceAnglesUnits=deg  RotationMatrix=[1 0 0; 0 1 0; 0 0 1]
  Rigid Transform1 : sm_lib/Frames and Transforms/Rigid Transform  TranslationMethod=StandardAxis  TranslationStandardOffset=h/2  TranslationLengthUnit=m  TranslationStandardAxis=+Z  TranslationCartesianOffset=[0 0 0]  TranslationROffset=0  TranslationROffsetUnits=m  TranslationZOffset=0  TranslationZOffsetUnits=m  TranslationThetaOffset=0  TranslationThetaOffsetUnits=deg  RotationMethod=None  RotationAngleUnits=deg  RotationStandardAxis=+Z  RotationAngle=0.0  RotationArbitraryAxis=[0 0 1]  FollAlignAxisA=+X  BaseAlignAxisA=+Y  FollAlignAxisB=+Y  BaseAlignAxisB=+Z  RotationSequenceAxes=FollowerAxes  RotationSequence=XYX  RotationSequenceAngles=[0 0 0]  RotationSequenceAnglesUnits=deg  RotationMatrix=[1 0 0; 0 1 0; 0 0 1]
  Solid : sm_lib/Body Elements/Brick Solid  GraphicAmbientColor=[0.15 0.15 0.15 1.0]  BasedOnType=Density  BrickDimensions=[d w h]  BrickDimensionUnits=m  CenterOfMass=[0 0 0]  CenterOfMassUnits=m  GraphicDiffuseColor=[0.2 0.8 1.0]  Density=rho  DensityUnits=kg/(m^3)  DoExposeReferenceFrame=on  GraphicEmissiveColor=[0.0 0.0 0.0 1.0]  ExportEntireGeometry=off  SerializedFrames=<Frames/>  MarkerShape=Sphere  MarkerSize=10  GraphicType=FromGeometry  InertiaType=CalculateFromGeometry  Mass=1  MassUnits=kg  MomentsOfInertia=[1 1 1]  MomentsOfInertiaUnits=kg*m^2  GraphicOpacity=1.0  ProductsOfInertia=[0 0 0]  ProductsOfInertiaUnits=kg*m^2  GraphicShininess=75  GraphicSpecularColor=[0.5 0.5 0.5 1.0]  GraphicVisPropType=SimpleVisualProperties
  Spline : sm_lib/Curves and Surfaces/Spline  GraphicAmbientColor=[0.15 0.15 0.15 1.0]  GraphicDiffuseColor=[0.0 1.0 0.0]  DataPoints=[0 0 0; -aa -aa 0]  DataPointsUnits=m  GraphicEmissiveColor=[0.0 0.0 0.0 1.0]  EndConditionType=Natural  MarkerShape=Sphere  MarkerSize=10  GraphicType=FromGeometry  GraphicOpacity=0.8  GraphicShininess=75  GraphicSpecularColor=[0.5 0.5 0.5 1.0]  GraphicVisPropType=SimpleVisualProperties
      settings: SourceProductName=Simscape Multibody
  Spline1 : sm_lib/Curves and Surfaces/Spline  GraphicAmbientColor=[0.15 0.15 0.15 1.0]  GraphicDiffuseColor=[0.0 1 0.0]  DataPoints=[-aa -aa 0; aa -aa 0]  DataPointsUnits=m  GraphicEmissiveColor=[0.0 0.0 0.0 1.0]  EndConditionType=Natural  MarkerShape=Frame  MarkerSize=10  GraphicType=FromGeometry  GraphicOpacity=0.8  GraphicShininess=75  GraphicSpecularColor=[0.5 0.5 0.5 1.0]  GraphicVisPropType=SimpleVisualProperties
      settings: SourceProductName=Simscape Multibody
  Spline2 : sm_lib/Curves and Surfaces/Spline  GraphicAmbientColor=[0.15 0.15 0.15 1.0]  GraphicDiffuseColor=[0.0 1 0.0]  DataPoints=[aa -aa 0; aa/2 -aa/2 0]  DataPointsUnits=m  GraphicEmissiveColor=[0.0 0.0 0.0 1.0]  EndConditionType=Natural  MarkerShape=Frame  MarkerSize=10  GraphicType=FromGeometry  GraphicOpacity=0.8  GraphicShininess=75  GraphicSpecularColor=[0.5 0.5 0.5 1.0]  GraphicVisPropType=SimpleVisualProperties
      settings: SourceProductName=Simscape Multibody
  Spline3 : sm_lib/Curves and Surfaces/Spline  GraphicAmbientColor=[0.15 0.15 0.15 1.0]  GraphicDiffuseColor=[0.0 1 0.0]  DataPoints=[aa/2 -aa/2 0; aa/2 aa/2 0]  DataPointsUnits=m  GraphicEmissiveColor=[0.0 0.0 0.0 1.0]  EndConditionType=Natural  MarkerShape=Frame  MarkerSize=10  GraphicType=FromGeometry  GraphicOpacity=0.8  GraphicShininess=75  GraphicSpecularColor=[0.5 0.5 0.5 1.0]  GraphicVisPropType=SimpleVisualProperties
      settings: SourceProductName=Simscape Multibody
  Spline4 : sm_lib/Curves and Surfaces/Spline  GraphicAmbientColor=[0.15 0.15 0.15 1.0]  GraphicDiffuseColor=[0.0 1 0.0]  DataPoints=[aa/2 aa/2 0; aa aa 0]  DataPointsUnits=m  GraphicEmissiveColor=[0.0 0.0 0.0 1.0]  EndConditionType=Natural  MarkerShape=Frame  MarkerSize=10  GraphicType=FromGeometry  GraphicOpacity=0.8  GraphicShininess=75  GraphicSpecularColor=[0.5 0.5 0.5 1.0]  GraphicVisPropType=SimpleVisualProperties
      settings: SourceProductName=Simscape Multibody
  Spline5 : sm_lib/Curves and Surfaces/Spline  GraphicAmbientColor=[0.15 0.15 0.15 1.0]  GraphicDiffuseColor=[0.0 1 0.0]  DataPoints=[aa aa 0; -aa aa 0]  DataPointsUnits=m  GraphicEmissiveColor=[0.0 0.0 0.0 1.0]  EndConditionType=Natural  MarkerShape=Frame  MarkerSize=10  GraphicType=FromGeometry  GraphicOpacity=0.8  GraphicShininess=75  GraphicSpecularColor=[0.5 0.5 0.5 1.0]  GraphicVisPropType=SimpleVisualProperties
      settings: SourceProductName=Simscape Multibody
  Spline6 : sm_lib/Curves and Surfaces/Spline  GraphicAmbientColor=[0.15 0.15 0.15 1.0]  GraphicDiffuseColor=[0.0 1 0.0]  DataPoints=[-aa aa 0; -aa/2 aa/2 0]  DataPointsUnits=m  GraphicEmissiveColor=[0.0 0.0 0.0 1.0]  EndConditionType=Natural  MarkerShape=Frame  MarkerSize=10  GraphicType=FromGeometry  GraphicOpacity=0.8  GraphicShininess=75  GraphicSpecularColor=[0.5 0.5 0.5 1.0]  GraphicVisPropType=SimpleVisualProperties
      settings: SourceProductName=Simscape Multibody
  Spline7 : sm_lib/Curves and Surfaces/Spline  GraphicAmbientColor=[0.15 0.15 0.15 1.0]  GraphicDiffuseColor=[0.0 1 0.0]  DataPoints=[-aa/2 aa/2 0; -aa/2 0 0]  DataPointsUnits=m  GraphicEmissiveColor=[0.0 0.0 0.0 1.0]  EndConditionType=Natural  MarkerShape=Frame  MarkerSize=10  GraphicType=FromGeometry  GraphicOpacity=0.8  GraphicShininess=75  GraphicSpecularColor=[0.5 0.5 0.5 1.0]  GraphicVisPropType=SimpleVisualProperties
      settings: SourceProductName=Simscape Multibody
  "[-aa -aa 0]" : sm_lib/Frames and Transforms/Rigid Transform  TranslationMethod=Cartesian  TranslationStandardOffset=w/2  TranslationLengthUnit=m  TranslationStandardAxis=+Y  TranslationCartesianOffset=[-aa -aa 0]  TranslationROffset=0  TranslationROffsetUnits=m  TranslationZOffset=0  TranslationZOffsetUnits=m  TranslationThetaOffset=0  TranslationThetaOffsetUnits=deg  RotationMethod=None  RotationAngleUnits=deg  RotationStandardAxis=+Z  RotationAngle=0  RotationArbitraryAxis=[0 0 1]  FollAlignAxisA=+Z  BaseAlignAxisA=-X  FollAlignAxisB=+X  BaseAlignAxisB=+Y  RotationSequenceAxes=FollowerAxes  RotationSequence=XYX  RotationSequenceAngles=[0 0 0]  RotationSequenceAnglesUnits=deg  RotationMatrix=[1 0 0; 0 1 0; 0 0 1]
  "[0 0 0]" : sm_lib/Frames and Transforms/Rigid Transform  TranslationMethod=Cartesian  TranslationStandardOffset=w/2  TranslationLengthUnit=m  TranslationStandardAxis=+Y  TranslationCartesianOffset=[0 0 0]  TranslationROffset=0  TranslationROffsetUnits=m  TranslationZOffset=0  TranslationZOffsetUnits=m  TranslationThetaOffset=0  TranslationThetaOffsetUnits=deg  RotationMethod=None  RotationAngleUnits=deg  RotationStandardAxis=+Z  RotationAngle=0  RotationArbitraryAxis=[0 0 1]  FollAlignAxisA=+Z  BaseAlignAxisA=-X  FollAlignAxisB=+X  BaseAlignAxisB=+Y  RotationSequenceAxes=FollowerAxes  RotationSequence=XYX  RotationSequenceAngles=[0 0 0]  RotationSequenceAnglesUnits=deg  RotationMatrix=[1 0 0; 0 1 0; 0 0 1]
  "[aa -aa 0]" : sm_lib/Frames and Transforms/Rigid Transform  TranslationMethod=Cartesian  TranslationStandardOffset=w/2  TranslationLengthUnit=m  TranslationStandardAxis=+Y  TranslationCartesianOffset=[aa -aa 0]  TranslationROffset=0  TranslationROffsetUnits=m  TranslationZOffset=0  TranslationZOffsetUnits=m  TranslationThetaOffset=0  TranslationThetaOffsetUnits=deg  RotationMethod=None  RotationAngleUnits=deg  RotationStandardAxis=+Z  RotationAngle=0  RotationArbitraryAxis=[0 0 1]  FollAlignAxisA=+Z  BaseAlignAxisA=-X  FollAlignAxisB=+X  BaseAlignAxisB=+Y  RotationSequenceAxes=FollowerAxes  RotationSequence=XYX  RotationSequenceAngles=[0 0 0]  RotationSequenceAnglesUnits=deg  RotationMatrix=[1 0 0; 0 1 0; 0 0 1]
  inertia from geometry1 : sm_lib/Body Elements/Brick Solid  GraphicAmbientColor=[0.15 0.15 0.15 1.0]  BasedOnType=Density  BrickDimensions=2*[h h h]  BrickDimensionUnits=m  CenterOfMass=[d/2 w/2 h/2]  CenterOfMassUnits=m  GraphicDiffuseColor=[0.0 0.4 0.2]  Density=900  DensityUnits=kg/(m^3)  DoExposeReferenceFrame=on  GraphicEmissiveColor=[0.0 0.0 0.0 1.0]  ExportEntireGeometry=off  SerializedFrames=<Frames/>  MarkerShape=Sphere  MarkerSize=10  GraphicType=FromGeometry  InertiaType=CalculateFromGeometry  Mass=m  MassUnits=kg  MomentsOfInertia=[1 1 Izz]  MomentsOfInertiaUnits=kg*m^2  GraphicOpacity=0.8  ProductsOfInertia=[0 0 0]  ProductsOfInertiaUnits=kg*m^2  GraphicShininess=75  GraphicSpecularColor=[0.5 0.5 0.5 1.0]  GraphicVisPropType=SimpleVisualProperties
  inertia from geometry2 : sm_lib/Body Elements/Brick Solid  GraphicAmbientColor=[0.15 0.15 0.15 1.0]  BasedOnType=Density  BrickDimensions=2*[h h h]  BrickDimensionUnits=m  CenterOfMass=[d/2 w/2 h/2]  CenterOfMassUnits=m  GraphicDiffuseColor=[0.0 0.4 0.2]  Density=900  DensityUnits=kg/(m^3)  DoExposeReferenceFrame=on  GraphicEmissiveColor=[0.0 0.0 0.0 1.0]  ExportEntireGeometry=off  SerializedFrames=<Frames/>  MarkerShape=Sphere  MarkerSize=10  GraphicType=FromGeometry  InertiaType=CalculateFromGeometry  Mass=m  MassUnits=kg  MomentsOfInertia=[1 1 Izz]  MomentsOfInertiaUnits=kg*m^2  GraphicOpacity=0.8  ProductsOfInertia=[0 0 0]  ProductsOfInertiaUnits=kg*m^2  GraphicShininess=75  GraphicSpecularColor=[0.5 0.5 0.5 1.0]  GraphicVisPropType=SimpleVisualProperties
  inertia from geometry3 : sm_lib/Body Elements/Brick Solid  GraphicAmbientColor=[0.15 0.15 0.15 1.0]  BasedOnType=Density  BrickDimensions=2*[h h h]  BrickDimensionUnits=m  CenterOfMass=[d/2 w/2 h/2]  CenterOfMassUnits=m  GraphicDiffuseColor=[0.0 0.4 0.2]  Density=900  DensityUnits=kg/(m^3)  DoExposeReferenceFrame=on  GraphicEmissiveColor=[0.0 0.0 0.0 1.0]  ExportEntireGeometry=off  SerializedFrames=<Frames/>  MarkerShape=Sphere  MarkerSize=10  GraphicType=FromGeometry  InertiaType=CalculateFromGeometry  Mass=m  MassUnits=kg  MomentsOfInertia=[1 1 Izz]  MomentsOfInertiaUnits=kg*m^2  GraphicOpacity=0.8  ProductsOfInertia=[0 0 0]  ProductsOfInertiaUnits=kg*m^2  GraphicShininess=75  GraphicSpecularColor=[0.5 0.5 0.5 1.0]  GraphicVisPropType=SimpleVisualProperties
  Top : PMIOPort  Side=Right
  World : PMIOPort  Port=2  Side=Left
  connections:
  World/RConn1 -- Rigid Transform/RConn1
  Rigid Transform/LConn1 -- Solid/RConn1 -- Reference Frame/RConn1 -- Rigid Transform1/LConn1
  Top/RConn1 -- "[0 0 0]"/LConn1 -- "[aa -aa 0]"/LConn1 -- "[-aa -aa 0]"/LConn1 -- Rigid Transform1/RConn1
  Graphic2/RConn1 -- Spline7/LConn1 -- Spline6/LConn1 -- Spline5/LConn1 -- Spline4/LConn1 -- Spline3/LConn1 -- Spline2/LConn1 -- Spline1/LConn1 -- Spline/LConn1 -- "[0 0 0]"/RConn1
  Graphic1/RConn1 -- "[-aa -aa 0]"/RConn1
  Graphic3/RConn1 -- "[aa -aa 0]"/RConn1

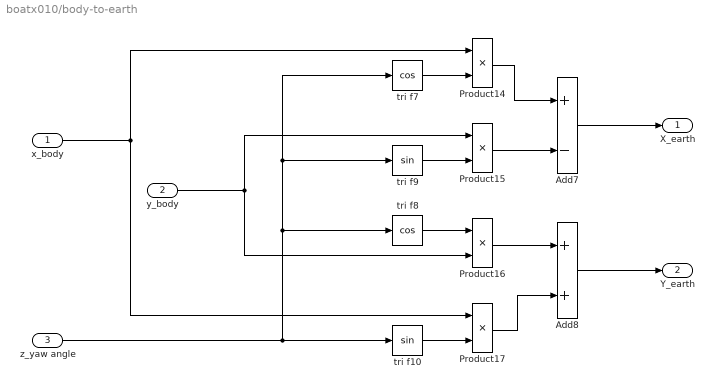
== system boatx010/body-to-earth ==
  x_body : Inport
  y_body : Inport  Port=2
  z_yaw angle : Inport  Port=3
  Add7 : Sum  Inputs=+-
  Add8 : Sum
  Product{14..17} (4 alike) : Product
  tri f10 : Trigonometry
  tri f7 : Trigonometry  Operator=cos
  tri f8 : Trigonometry  Operator=cos
  tri f9 : Trigonometry
  X_earth : Outport  VectorParamsAs1DForOutWhenUnconnected=off
  Y_earth : Outport  Port=2  VectorParamsAs1DForOutWhenUnconnected=off
  wires:
  tri f7/1 -> Product14/2
  tri f10/1 -> Product17/2
  y_body/1 -> Product16/2, Product15/1
  tri f9/1 -> Product15/2
  Add7/1 -> X_earth/1
  tri f8/1 -> Product16/1
  Product17/1 -> Add8/2
  Product15/1 -> Add7/2
  Add8/1 -> Y_earth/1
  Product16/1 -> Add8/1
  Product14/1 -> Add7/1
  z_yaw angle/1 -> tri f7/1, tri f9/1, tri f8/1, tri f10/1
  x_body/1 -> Product17/1, Product14/1

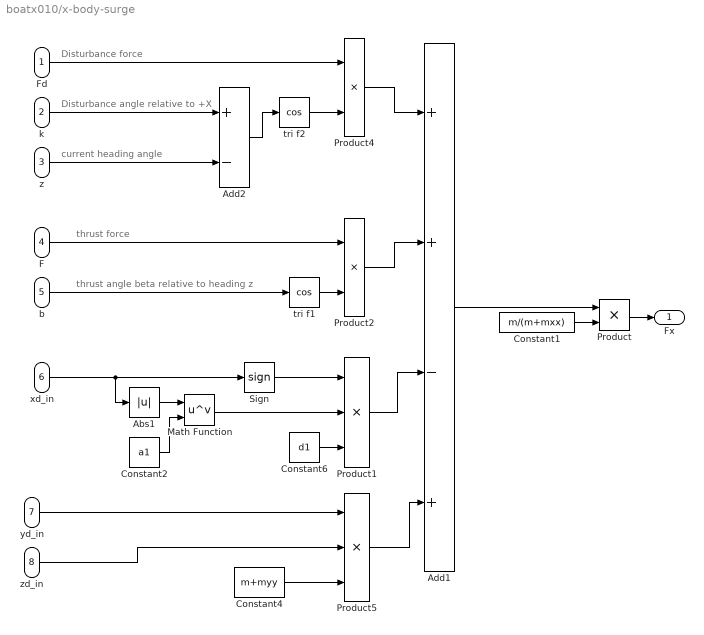
== system boatx010/x-body-surge ==
  note: current heading angle
  note: thrust force
  note: thrust angle beta relative to heading z
  note: Disturbance force
  note: Disturbance angle relative to +X
  Fd : Inport
  k : Inport  Port=2
  z : Inport  Port=3
  F : Inport  Port=4
  b : Inport  Port=5
  xd_in : Inport  Port=6
  yd_in : Inport  Port=7
  zd_in : Inport  Port=8
  Abs1 : Abs
  Add1 : Sum  Inputs=++-+
  Add2 : Sum  Inputs=+-
  Constant1 : Constant  Value=m/(m+mxx)
  Constant2 : Constant  Value=a1
  Constant4 : Constant  Value=m+myy  VectorParams1D=off
  Constant6 : Constant  Value=d1
  Math Function : Math  Operator=pow  SaturateOnIntegerOverflow=on
  Product : Product
  Product1 : Product  Inputs=3
  Product2 : Product
  Product4 : Product
  Product5 : Product  Inputs=3
  Sign : Signum
  tri f1 : Trigonometry  Operator=cos
  tri f2 : Trigonometry  Operator=cos
  Fx : Outport  VectorParamsAs1DForOutWhenUnconnected=off
  wires:
  xd_in/1 -> Sign/1, Abs1/1
  tri f1/1 -> Product2/2
  b/1 -> tri f1/1
  F/1 -> Product2/1
  Product4/1 -> Add1/1
  tri f2/1 -> Product4/2
  Fd/1 -> Product4/1
  Product2/1 -> Add1/2
  Add2/1 -> tri f2/1
  k/1 -> Add2/1
  z/1 -> Add2/2
  Product5/1 -> Add1/4
  yd_in/1 -> Product5/1
  zd_in/1 -> Product5/2
  Constant4/1 -> Product5/3
  Product1/1 -> Add1/3
  Abs1/1 -> Math Function/1
  Constant2/1 -> Math Function/2
  Math Function/1 -> Product1/2
  Constant6/1 -> Product1/3
  Sign/1 -> Product1/1
  Product/1 -> Fx/1
  Add1/1 -> Product/1
  Constant1/1 -> Product/2

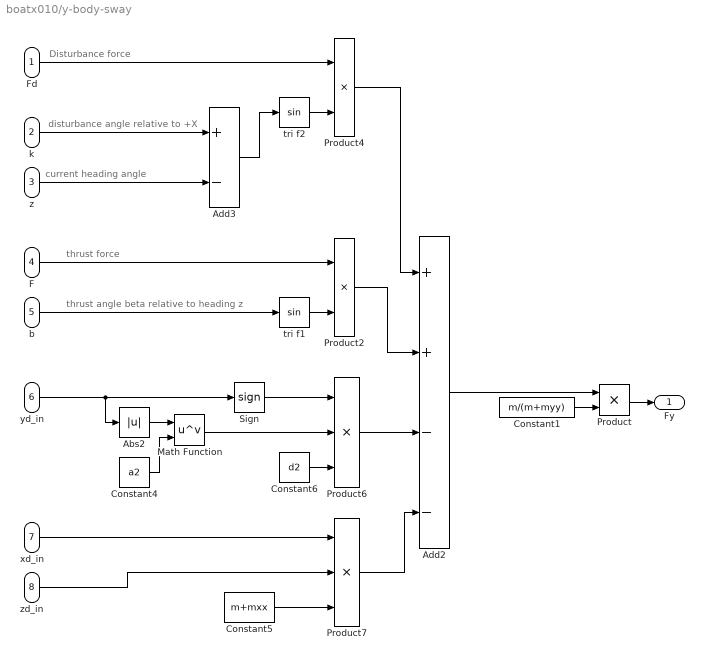
== system boatx010/y-body-sway ==
  note: thrust force
  note: thrust angle beta relative to heading z
  note: Disturbance force
  note: current heading angle
  note: disturbance angle relative to +X
  Fd : Inport
  k : Inport  Port=2
  z : Inport  Port=3
  F : Inport  Port=4
  b : Inport  Port=5
  yd_in : Inport  Port=6
  xd_in : Inport  Port=7
  zd_in : Inport  Port=8
  Abs2 : Abs
  Add2 : Sum  Inputs=++--
  Add3 : Sum  Inputs=+-
  Constant1 : Constant  Value=m/(m+myy)
  Constant4 : Constant  Value=a2
  Constant5 : Constant  Value=m+mxx  VectorParams1D=off
  Constant6 : Constant  Value=d2
  Math Function : Math  Operator=pow  SaturateOnIntegerOverflow=on
  Product : Product
  Product2 : Product
  Product4 : Product
  Product6 : Product  Inputs=3
  Product7 : Product  Inputs=3
  Sign : Signum
  tri f1 : Trigonometry
  tri f2 : Trigonometry
  Fy : Outport  VectorParamsAs1DForOutWhenUnconnected=off
  wires:
  Product2/1 -> Add2/2
  tri f1/1 -> Product2/2
  b/1 -> tri f1/1
  F/1 -> Product2/1
  Product4/1 -> Add2/1
  tri f2/1 -> Product4/2
  Fd/1 -> Product4/1
  k/1 -> Add3/1
  z/1 -> Add3/2
  Add3/1 -> tri f2/1
  yd_in/1 -> Sign/1, Abs2/1
  Product7/1 -> Add2/4
  xd_in/1 -> Product7/1
  zd_in/1 -> Product7/2
  Constant5/1 -> Product7/3
  Product6/1 -> Add2/3
  Abs2/1 -> Math Function/1
  Constant4/1 -> Math Function/2
  Math Function/1 -> Product6/2
  Constant6/1 -> Product6/3
  Sign/1 -> Product6/1
  Add2/1 -> Product/1
  Constant1/1 -> Product/2
  Product/1 -> Fy/1
